simulink model "book_2"  (R2016b)
settings: Solver=VariableStepAuto  StartTime=0.0  StopTime=10.0  RelTol=1e-3
settings Model: Creator=zbn02  LastModifiedBy=zbn02

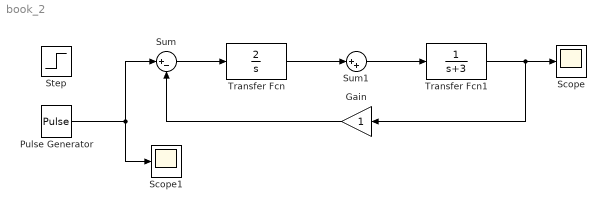
== system book_2 ==
  Gain : Gain
  Pulse Generator : DiscretePulseGenerator  PulseType=Time based  Period=10  PulseWidth=50
  Scope : Scope
  Scope1 : Scope
  Step : Step  SampleTime=0
  Sum : Sum  Inputs=|+-
  Sum1 : Sum  Inputs=|++
  Transfer Fcn : TransferFcn  Numerator=[2]  Denominator=[1 0]
  Transfer Fcn1 : TransferFcn  Denominator=[1 3]
  wires:
  Transfer Fcn1/1 -> Gain/1, Scope/1
  Sum1/1 -> Transfer Fcn1/1
  Transfer Fcn/1 -> Sum1/1
  Sum/1 -> Transfer Fcn/1
  Pulse Generator/1 -> Scope1/1, Sum/1
  Gain/1 -> Sum/2
